simulink model "sl_pursuit_2019b"  (R2019b)
settings: Solver=FixedStepAuto  StartTime=0.0  StopTime=20  FixedStep=0.05  MaxStep=0.05  RelTol=1e-3  EnableMultiTasking=on
StartFcn:
  | % remove the red dashed line draw in StopFcn
  | h = findobj('Tag',  'SL_PURSUIT_PATH');
  | if ~isempty(h)
  |     delete(h)
  | end
StopFcn:
  | % get the waypoints from trajectory block
  | h = getSimulinkBlockHandle([gcs '/trajectory'])
  | path = str2num(get_param(h, 'path'));
  | 
  | % overlay it on the XY scope, tag it so it can be cleaned up in StartFcn
  | set(0, 'ShowHiddenHandles', 'on')
  | hold on
  | plot(path(:,1), path(:,2), 'Color',  'red', 'LineStyle', '--', 'LineWidth', 2, 'Tag', 'SL_PURSUIT_PATH')
  | hold off
  | set(0, 'ShowHiddenHandles', 'on')
libraries: roblocks x2, simulink_need_slupdate x1, simulink x1
settings Model: EnablePacing=on  Creator=pic  LastModifiedBy=Jamie
settings DataIOCC: SaveFormat=Array  SignalLoggingSaveFormat=ModelDataLogs  TimeSaveName=t  OutputSaveName=y
settings OptimizationCC: ExpressionDepthLimit=2147483647  LifeSpan=inf
settings DebuggingCC: UnderspecifiedInitializationDetection=Classic  MergeDetectMultiDrivingBlocksExec=none  SolverPrmCheckMsg=warning  FcnCallInpInsideContextMsg=warning  AllowSymbolicDim=off  StateNameClashWarn=warning  SFUnexpectedBacktrackingDiag=warning  SFNoUnconditionalDefaultTransitionDiag=warning  SFExecutionAtInitializationDiag=none  ArithmeticOperatorsInVariantConditions=warning
settings HardwareCC: ProdBitPerPointer=32  ProdBitPerSizeT=32  ProdBitPerPtrDiffT=32  ProdLargestAtomicFloat=None  ProdIntDivRoundTo=Undefined  ProdEndianess=Unspecified  ProdWordSize=32  ProdHWDeviceType=32-bit Generic
settings ModelReferenceCC: PropagateSignalLabelsOutOfModel=off
settings SFSimCC: SimUseLocalCustomCode=off  CustomCodeUndefinedFunction=UseInterfaceOnly
settings RTWCC: RTWUseLocalCustomCode=off
settings CodeAppCC: StateflowObjectComments=on
settings GRTTargetCC: TargetLangStandard=C89/C90 (ANSI)  CombineOutputUpdateFcns=off  GRTInterface=on
settings ConfigComp: CovMetricSettings=dw  CovHtmlReporting=on  CovSaveCumulativeToWorkspaceVar=on  CovSaveSingleToWorkspaceVar=on  CovExternalEMLEnable=off

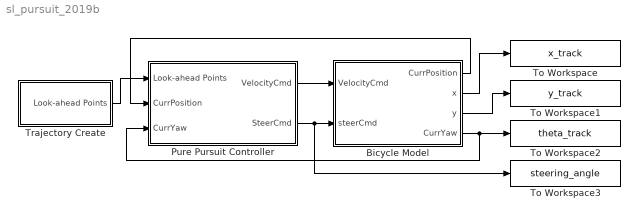
== system sl_pursuit_2019b ==
  Bicycle Model : Subsystem
  Pure Pursuit Controller : Subsystem
  To Workspace : ToWorkspace  VariableName=x_track  SampleTime=-1
      settings: Save2DSignal=2-D array (concatenate along first dimension)
  To Workspace1 : ToWorkspace  VariableName=y_track  SampleTime=-1
      settings: Save2DSignal=2-D array (concatenate along first dimension)
  To Workspace2 : ToWorkspace  VariableName=theta_track  SampleTime=-1
      settings: Save2DSignal=2-D array (concatenate along first dimension)
  To Workspace3 : ToWorkspace  VariableName=steering_angle  SampleTime=-1
      settings: Save2DSignal=2-D array (concatenate along first dimension)
  Trajectory Create : Subsystem
  wires:
  Bicycle Model/4(CurrYaw) -> Pure Pursuit Controller/3(CurrYaw), To Workspace2/1
  Bicycle Model/2(x) -> To Workspace/1
  Bicycle Model/3(y) -> To Workspace1/1
  Pure Pursuit Controller/2(SteerCmd) -> To Workspace3/1, Bicycle Model/2(steerCmd)
  Trajectory Create/1(Look-ahead Points) -> Pure Pursuit Controller/1(Look-ahead Points)
  Bicycle Model/1(CurrPosition) -> Pure Pursuit Controller/2(CurrPosition)
  Pure Pursuit Controller/1(VelocityCmd) -> Bicycle Model/1(VelocityCmd)

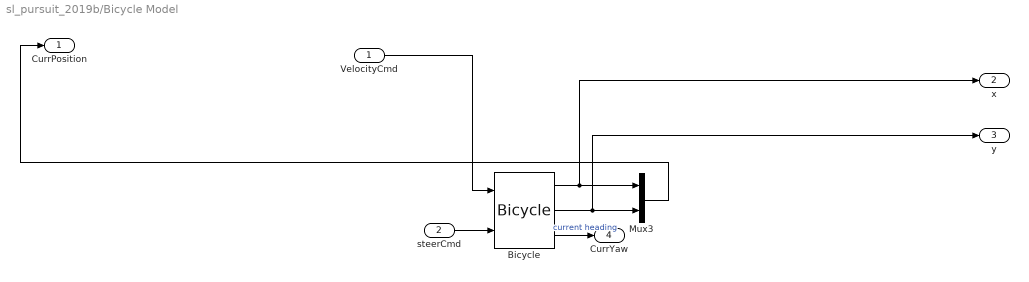
== system sl_pursuit_2019b/Bicycle Model ==
  VelocityCmd : Inport
  steerCmd : Inport  Port=2
  Bicycle : roblocks/Vehicles/Bicycle  vlim=5  accel=1  alim=0.5  steer_rate=Inf  L=0.324  x0=[0, 0, 1.5707]
      link override acceleration limit: RisingSlewLimit=3  FallingSlewLimit=-3
      link override steering angle limit: UpperLimit=3  LowerLimit=-3
      link override steering rate limit: RisingSlewLimit=3  FallingSlewLimit=-3
      link override vel limit: UpperLimit=3  LowerLimit=-3
  Mux3 : Mux  Inputs=2
  CurrPosition : Outport
  x : Outport  Port=2
  y : Outport  Port=3
  CurrYaw : Outport  Port=4
  wires:
  Mux3/1 -> CurrPosition/1
  Bicycle/1 -> x/1, Mux3/1
  steerCmd/1 -> Bicycle/2
  VelocityCmd/1 -> Bicycle/1
  Bicycle/2 -> y/1, Mux3/2
  Bicycle/3 -> CurrYaw/1  "current heading"

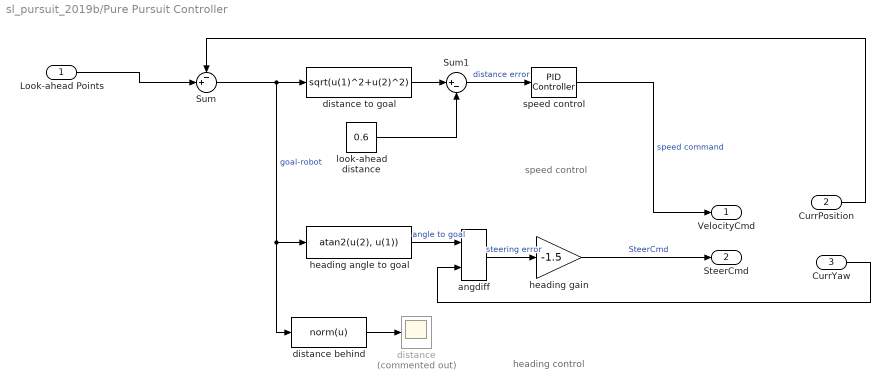
== system sl_pursuit_2019b/Pure Pursuit Controller ==
  note: speed control
  note: heading control
  Look-ahead Points : Inport
  CurrPosition : Inport  Port=2
  CurrYaw : Inport  Port=3
  Sum : Sum  Inputs=-+|
  Sum1 : Sum  Inputs=|+-
  angdiff : roblocks/Toolbox/angdiff
  distance : Scope  Commented=on
  distance behind : MATLABFcn  MATLABFcn=norm(u)
  distance to goal : Fcn  Expr=sqrt(u(1)^2+u(2)^2)
  heading angle to goal : Fcn  Expr=atan2(u(2), u(1))
  heading gain : Gain  Gain=-1.5
  look-ahead distance : Constant  Value=0.6
  speed control : simulink_need_slupdate/PID Controller  P=1.5  I=1.62  D=0.12
  VelocityCmd : Outport
  SteerCmd : Outport  Port=2
  wires:
  CurrPosition/1 -> Sum/1
  heading angle to goal/1 -> angdiff/1  "angle to goal"
  Sum/1 -> distance behind/1, heading angle to goal/1, distance to goal/1  "goal-robot"
  distance to goal/1 -> Sum1/1
  speed control/1 -> VelocityCmd/1  "speed command"
  Sum1/1 -> speed control/1  "distance error"
  angdiff/1 -> heading gain/1  "steering error"
  look-ahead distance/1 -> Sum1/2
  distance behind/1 -> distance/1
  CurrYaw/1 -> angdiff/2
  heading gain/1 -> SteerCmd/1  "SteerCmd"
  Look-ahead Points/1 -> Sum/2

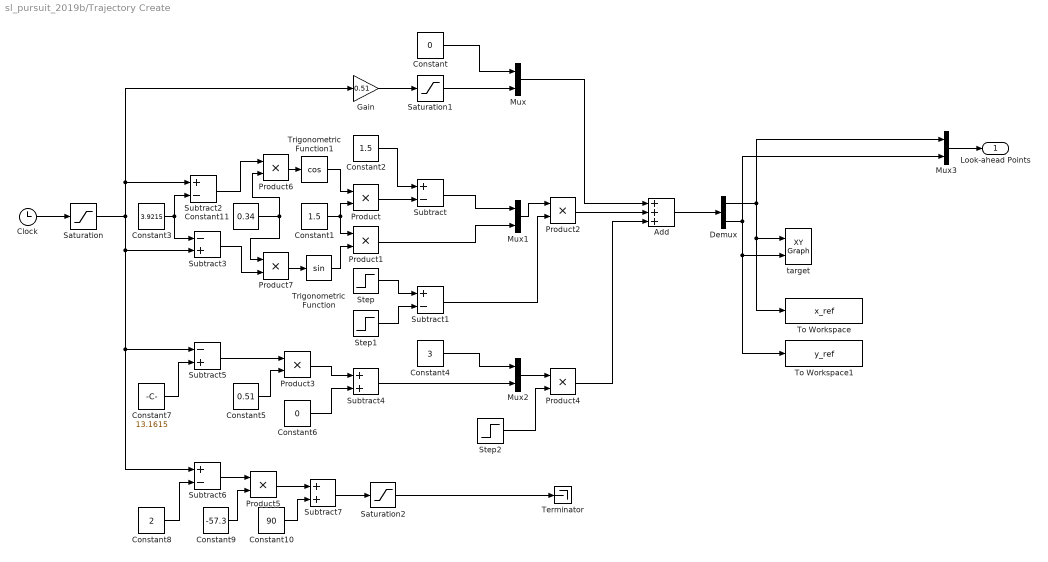
== system sl_pursuit_2019b/Trajectory Create ==
  Add : Sum  Inputs=+++
  Clock : Clock
  Constant : Constant  Value=0
  Constant1 : Constant  Value=1.5
  Constant10 : Constant  Value=90
  Constant11 : Constant  Value=0.34
  Constant2 : Constant  Value=1.5
  Constant3 : Constant  Value=3.9215
  Constant4 : Constant  Value=3
  Constant5 : Constant  Value=0.51
  Constant6 : Constant  Value=0
  Constant7 : Constant  Value=13.1615
  Constant8 : Constant  Value=2
  Constant9 : Constant  Value=-57.3
  Demux : Demux  Outputs=2
  Gain : Gain  Gain=0.51
  Mux{,1..3} (4 alike) : Mux  Inputs=2
  Product{,1..7} (8 alike) : Product
  Saturation : Saturate  UpperLimit=18  LowerLimit=0
  Saturation1 : Saturate  UpperLimit=2  LowerLimit=0
  Saturation2 : Saturate  UpperLimit=90  LowerLimit=-90
  Step : Step  Time=3.9216  SampleTime=0
  Step1 : Step  Time=13.1615  SampleTime=0
  Step2 : Step  Time=13.1615  SampleTime=0
  Subtract{,1..2,6} (4 alike) : Sum  Inputs=+-
  Subtract3 : Sum  Inputs=-+
  Subtract4 : Sum
  Subtract5 : Sum  Inputs=-+
  Subtract7 : Sum
  Terminator : Terminator
  To Workspace : ToWorkspace  VariableName=x_ref  SampleTime=-1
      settings: Save2DSignal=2-D array (concatenate along first dimension)
  To Workspace1 : ToWorkspace  VariableName=y_ref  SampleTime=-1
      settings: Save2DSignal=2-D array (concatenate along first dimension)
  Trigonometric Function : Trigonometry
  Trigonometric Function1 : Trigonometry  Operator=cos
  target : simulink/Sinks/XY Graph  xmin=-1  xmax=5  ymin=-1  ymax=5  st=-1
  Look-ahead Points : Outport  VectorParamsAs1DForOutWhenUnconnected=off
  wires:
  Clock/1 -> Saturation/1
  Add/1 -> Demux/1
  Mux/1 -> Add/1
  Constant/1 -> Mux/1
  Saturation1/1 -> Mux/2
  Gain/1 -> Saturation1/1
  Demux/1 -> Mux3/1, To Workspace/1, target/1
  Demux/2 -> Mux3/2, To Workspace1/1, target/2
  Trigonometric Function1/1 -> Product/1
  Trigonometric Function/1 -> Product1/2
  Constant1/1 -> Product1/1, Product/2
  Product/1 -> Subtract/2
  Constant2/1 -> Subtract/1
  Subtract/1 -> Mux1/1
  Product1/1 -> Mux1/2
  Step/1 -> Subtract1/1
  Step1/1 -> Subtract1/2
  Subtract1/1 -> Product2/2
  Mux1/1 -> Product2/1
  Product2/1 -> Add/2
  Constant3/1 -> Subtract3/1, Subtract2/2
  Constant4/1 -> Mux2/1
  Constant5/1 -> Product3/2
  Product3/1 -> Subtract4/1
  Constant6/1 -> Subtract4/2
  Subtract4/1 -> Mux2/2
  Mux2/1 -> Product4/1
  Step2/1 -> Product4/2
  Product4/1 -> Add/3
  Constant7/1 -> Subtract5/2
  Saturation/1 -> Subtract6/1, Subtract5/1, Subtract3/2, Subtract2/1, Gain/1
  Subtract5/1 -> Product3/1
  Mux3/1 -> Look-ahead Points/1
  Constant8/1 -> Subtract6/2
  Subtract6/1 -> Product5/1
  Constant9/1 -> Product5/2
  Product5/1 -> Subtract7/1
  Constant10/1 -> Subtract7/2
  Subtract7/1 -> Saturation2/1
  Saturation2/1 -> Terminator/1
  Product6/1 -> Trigonometric Function1/1
  Product7/1 -> Trigonometric Function/1
  Subtract2/1 -> Product6/1
  Subtract3/1 -> Product7/2
  Constant11/1 -> Product6/2, Product7/1
